simulink model "scopeInterface_SS"  (R2023b)
settings: Solver=FixedStepAuto  StartTime=0.0  StopTime=30  FixedStep=0.01  RelTol=1e-3
undefined symbols (not defined in the file or in its folder): ka, kp, kv, param
settings Model: PacingRate=1.530000  Creator=Scott.Dahlke  LastModifiedBy=Connor Emmons
settings SolverCC: AlgebraicLoopSolver=TrustRegion
settings DebuggingCC: UnconnectedInputMsg=warning  UnconnectedOutputMsg=warning  UnconnectedLineMsg=warning
settings ModelReferenceCC: EnableRefExpFcnMdlSchedulingChecks=on
settings SFSimCC: CustomCodeUndefinedFunction=UseInterfaceOnly
settings RTWCC: DLArmComputeVersion=19.05

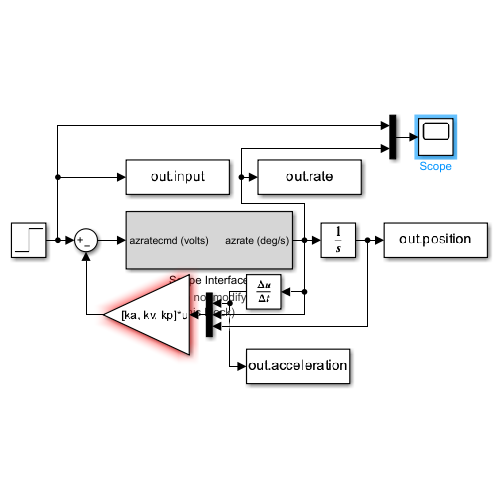
[thumbnail: Simulink's stored preview of the top-level diagram]
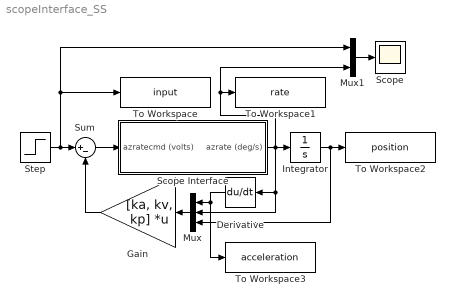
== system scopeInterface_SS ==
  Derivative : Derivative
  Gain : Gain  Gain=[ka, kv, kp]  Multiplication=Matrix(K*u)
  Integrator : Integrator
  Mux : Mux  Inputs=3
  Mux1 : Mux  Inputs=2
  Scope : Scope
  Scope Interface : Subsystem
      settings: AttributesFormatString=|
      | (Do not modify
      | this block)
  Step : Step  SampleTime=0
  Sum : Sum  Inputs=|+-
  To Workspace : ToWorkspace  VariableName=input  SampleTime=-1
  To Workspace1 : ToWorkspace  VariableName=rate  SampleTime=-1
  To Workspace2 : ToWorkspace  VariableName=position  SampleTime=-1
  To Workspace3 : ToWorkspace  VariableName=acceleration  SampleTime=-1
  wires:
  Scope Interface/1(azrate (deg/s)) -> Mux1/2, To Workspace1/1, Mux/2, Derivative/1, Integrator/1
  Sum/1 -> Scope Interface/1(azratecmd (volts))
  Step/1 -> Mux1/1, To Workspace/1, Sum/1
  Derivative/1 -> To Workspace3/1, Mux/1
  Mux/1 -> Gain/1
  Gain/1 -> Sum/2
  Integrator/1 -> Mux/3, To Workspace2/1
  Mux1/1 -> Scope/1

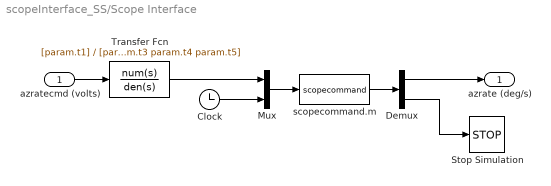
== system scopeInterface_SS/Scope Interface ==
  azratecmd (volts) : Inport
  Clock : Clock
  Demux : Demux  Outputs=2
  Mux : Mux  Inputs=2
  Stop Simulation : Stop
  Transfer Fcn : TransferFcn  Numerator=[param.t1]  Denominator=[param.t3 param.t4 param.t5]
  scopecommand.m : MATLABFcn  MATLABFcn=scopecommand  OutputDimensions=2
  azrate (deg/s) : Outport
  wires:
  azratecmd (volts)/1 -> Transfer Fcn/1
  Mux/1 -> scopecommand.m/1
  Demux/2 -> Stop Simulation/1
  Demux/1 -> azrate (deg/s)/1
  scopecommand.m/1 -> Demux/1
  Transfer Fcn/1 -> Mux/1
  Clock/1 -> Mux/2
